simulink model "k1visitmxmon"  (Simulink 8.6)
settings: Solver=VariableStepAuto  StartTime=0.0  StopTime=10.0  RelTol=1e-3
libraries: cdsAdcx0 x1, cdsAdcx1 x1, cdsAdcx2 x1, VISMON_MASTER x1, cdsIPCx x1, cdsModelRate x1, cdsParameters x1
settings Model: Creator=controls  LastModifiedBy=controls
settings DataIOCC: SaveFormat=Dataset  SignalLoggingSaveFormat=Dataset
settings OptimizationCC: ExpressionDepthLimit=128
settings DebuggingCC: UnderspecifiedInitializationDetection=Simplified  MergeDetectMultiDrivingBlocksExec=error  SolverPrmCheckMsg=none  FcnCallInpInsideContextMsg=EnableAllAsError  StateNameClashWarn=none
settings HardwareCC: ProdBitPerPointer=64  ProdLargestAtomicFloat=Float  ProdIntDivRoundTo=Zero  ProdEndianess=LittleEndian  ProdWordSize=64  ProdHWDeviceType=Intel->x86-64 (Windows64)
settings GRTTargetCC: GeneratePreprocessorConditionals=Use local settings  CombineOutputUpdateFcns=on  GRTInterface=off
settings ConfigComp: CovModelRefEnable=off

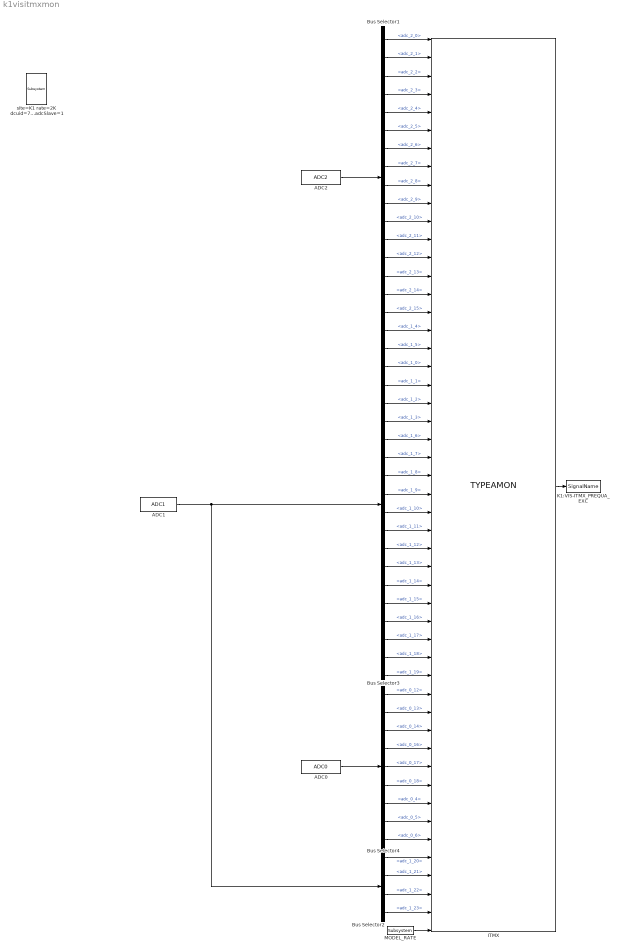
== system k1visitmxmon ==
  ADC0 : cdsAdcx0/ADC0  Tag=cdsAdc  Description=|
      | type-GSC_16AI64SSA
      | card_num=0
      settings: AttributesFormatString=%<Description>\n%<Tag>
  ADC1 : cdsAdcx1/ADC1  Tag=cdsAdc  Description=|
      | type-GSC_16AI64SSA
      | card_num=1
      settings: AttributesFormatString=%<Description>\n%<Tag>
  ADC2 : cdsAdcx2/ADC2  Tag=cdsAdc  Description=|
      | type-GSC_16AI64SSA
      | card_num=2
      settings: AttributesFormatString=%<Description>\n%<Tag>
  Bus Selector1 : BusSelector  Description=ADC Selector  OutputSignals=adc_2_0,adc_2_1,adc_2_2,adc_2_3,adc_2_4,adc_2_5,adc_2_6,adc_2_7,adc_2_8,adc_2_9,adc_2_10,adc_2_11,adc_2_12,adc_2_13,adc_2_14,adc_2_15
      settings: AttributesFormatString=%<Description>
  Bus Selector2 : BusSelector  OutputSignals=adc_1_20,adc_1_21,adc_1_22,adc_1_23
  Bus Selector3 : BusSelector  OutputSignals=adc_1_4,adc_1_5,adc_1_0,adc_1_1,adc_1_2,adc_1_3,adc_1_6,adc_1_7,adc_1_8,adc_1_9,adc_1_10,adc_1_11,adc_1_12,adc_1_13,adc_1_14,adc_1_15,adc_1_16,adc_1_17,adc_1_18,adc_1_19
  Bus Selector4 : BusSelector  OutputSignals=adc_0_12,adc_0_13,adc_0_14,adc_0_16,adc_0_17,adc_0_18,adc_0_4,adc_0_5,adc_0_6
  ITMX : VISMON_MASTER/TYPEAMON
  K1:VIS-ITMX_PREQUA_EXC : cdsIPCx/SignalName  Tag=cdsIPCx_SHMEM  Description=Inter-Process Communication via Shared memory.
      settings: AttributesFormatString=%<Tag>
  MODEL_RATE : cdsModelRate/Subsystem  Tag=cdsModelRate
      settings: AttributesFormatString=%<Tag>
  site=K1 rate=2K dcuid=77 host=k1ix1 specific_cpu=1 adcSlave=1 : cdsParameters/Subsystem  Tag=cdsParameters  Description=|
      | Purpose:                                                                                                                                                                                                                                
      | Provide system parameters to the FE code generator to properly configure the generated EPICS names, rep rate of the FE controller, and the Data Acquisition node ID for proper storage of data from this FE controller.                 
      |                                                                                                                                                                                                                                         
      | Useage:                                                                                                                                                                                                                                 
      | The part NAME field is used to identify the FE parameters. It must be of the form:                                                                                                                                                      
      | site=                                                                                                                                                                                                                                   
      | rate=                                                                                                                                                                                                                                   
      | dcuid=                                                                                                                                                                                                                                  
      |                                                                                                                                                                                                                                         
      | Where:                                                                                                                                                                                                                                  
      | site= argument may be H1, H2, L1, M1, G1, either as a single argument or multiple, for example site=H1,H2. These are the only names allowed. These will become the first two characters of all EPICS and signal names (for example G1:).
      |                                                                                                                                                                                                                                         
      | rate= may be 2K, 16K, 32K, or 64K                                                                                                                                                                                                       
      |                                                                                                                                                                                                                                         
      | dcuid= is site specific ie it must be unique at each site.
      settings: AttributesFormatString=%<Tag>
  wires:
  ADC2/1 -> Bus Selector1/1
  Bus Selector1/1 -> ITMX/1  "<adc_2_0>"
  Bus Selector1/2 -> ITMX/2  "<adc_2_1>"
  Bus Selector1/3 -> ITMX/3  "<adc_2_2>"
  Bus Selector1/4 -> ITMX/4  "<adc_2_3>"
  Bus Selector1/5 -> ITMX/5  "<adc_2_4>"
  Bus Selector1/6 -> ITMX/6  "<adc_2_5>"
  Bus Selector1/7 -> ITMX/7  "<adc_2_6>"
  Bus Selector1/8 -> ITMX/8  "<adc_2_7>"
  Bus Selector1/9 -> ITMX/9  "<adc_2_8>"
  Bus Selector1/10 -> ITMX/10  "<adc_2_9>"
  Bus Selector1/11 -> ITMX/11  "<adc_2_10>"
  Bus Selector1/12 -> ITMX/12  "<adc_2_11>"
  Bus Selector1/13 -> ITMX/13  "<adc_2_12>"
  Bus Selector1/14 -> ITMX/14  "<adc_2_13>"
  Bus Selector1/15 -> ITMX/15  "<adc_2_14>"
  Bus Selector1/16 -> ITMX/16  "<adc_2_15>"
  MODEL_RATE/1 -> ITMX/50
  ITMX/1 -> K1:VIS-ITMX_PREQUA_EXC/1
  ADC1/1 -> Bus Selector2/1, Bus Selector3/1
  Bus Selector3/1 -> ITMX/17  "<adc_1_4>"
  Bus Selector3/2 -> ITMX/18  "<adc_1_5>"
  Bus Selector3/3 -> ITMX/19  "<adc_1_0>"
  Bus Selector3/4 -> ITMX/20  "<adc_1_1>"
  Bus Selector3/5 -> ITMX/21  "<adc_1_2>"
  Bus Selector3/6 -> ITMX/22  "<adc_1_3>"
  Bus Selector3/7 -> ITMX/23  "<adc_1_6>"
  Bus Selector3/8 -> ITMX/24  "<adc_1_7>"
  Bus Selector3/9 -> ITMX/25  "<adc_1_8>"
  Bus Selector3/10 -> ITMX/26  "<adc_1_9>"
  Bus Selector3/11 -> ITMX/27  "<adc_1_10>"
  Bus Selector3/12 -> ITMX/28  "<adc_1_11>"
  Bus Selector3/13 -> ITMX/29  "<adc_1_12>"
  Bus Selector3/14 -> ITMX/30  "<adc_1_13>"
  Bus Selector3/15 -> ITMX/31  "<adc_1_14>"
  Bus Selector3/16 -> ITMX/32  "<adc_1_15>"
  Bus Selector3/17 -> ITMX/33  "<adc_1_16>"
  Bus Selector3/18 -> ITMX/34  "<adc_1_17>"
  Bus Selector3/19 -> ITMX/35  "<adc_1_18>"
  Bus Selector3/20 -> ITMX/36  "<adc_1_19>"
  ADC0/1 -> Bus Selector4/1
  Bus Selector4/1 -> ITMX/37  "<adc_0_12>"
  Bus Selector4/2 -> ITMX/38  "<adc_0_13>"
  Bus Selector4/3 -> ITMX/39  "<adc_0_14>"
  Bus Selector4/4 -> ITMX/40  "<adc_0_16>"
  Bus Selector4/5 -> ITMX/41  "<adc_0_17>"
  Bus Selector4/6 -> ITMX/42  "<adc_0_18>"
  Bus Selector4/7 -> ITMX/43  "<adc_0_4>"
  Bus Selector4/8 -> ITMX/44  "<adc_0_5>"
  Bus Selector4/9 -> ITMX/45  "<adc_0_6>"
  Bus Selector2/1 -> ITMX/46  "<adc_1_20>"
  Bus Selector2/2 -> ITMX/47  "<adc_1_21>"
  Bus Selector2/3 -> ITMX/48  "<adc_1_22>"
  Bus Selector2/4 -> ITMX/49  "<adc_1_23>"
